simulink model "simulation"  (R2024a)
settings: Solver=FixedStepAuto  StartTime=0.0  StopTime=100  FixedStep=ts  RelTol=1e-3
values from neighbouring files (symbols this model uses):
  C = [0, 0, 1, 0, 0, 0 ... (first row only)    [setup.m]
  Ig = 10*(m*l^2)/3    (= 6)    [setup.m]
  m = 5    [setup.m]
  ni_r = 1    [setup.m]
  ni_x = 1    [setup.m]
  ni_y = 6    [setup.m]
  u_eq = [m*g; 0]    [setup.m]
  w = [1,      1 ... (first row only)    [setup.m]
  z_eq = z_init    [setup.m]
  z_init = [0;0;0;0;0;0]    [setup.m]
libraries: slpidlib x3, simulink x2
settings Model: Creator=enead  LastModifiedBy=enead
settings SolverCC: EnableFixedStepZeroCrossing=on
settings OptimizationCC: ReuseModelBlockBuffer=off
settings RTWCC: GPUComputeCapability=3.5

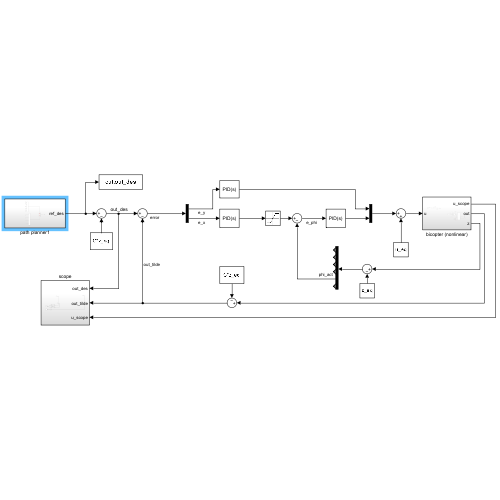
[thumbnail: Simulink's stored preview of the top-level diagram]
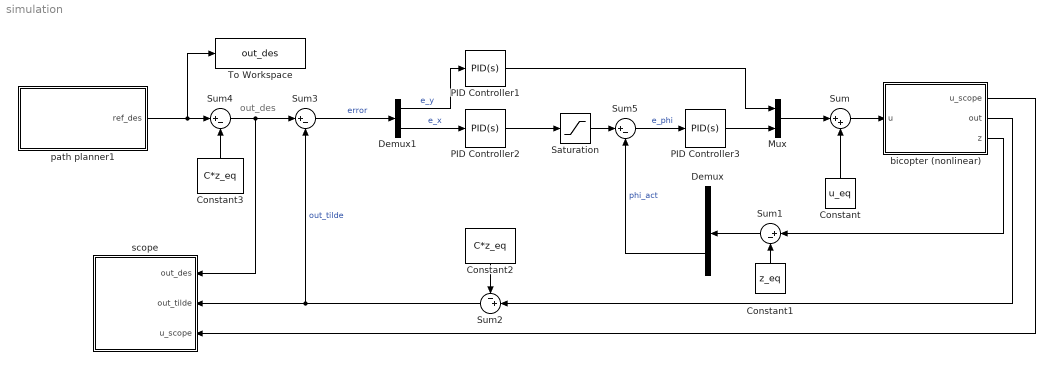
== system simulation ==
  note: out_des
  Constant : Constant  Value=u_eq
  Constant1 : Constant  Value=z_eq
  Constant2 : Constant  Value=C*z_eq
  Constant3 : Constant  Value=C*z_eq
  Demux : Demux  Outputs=6
  Demux1 : Demux  Outputs=2
  Mux : Mux  Inputs=2
  PID Controller1 : slpidlib/PID Controller  Controller=PID  Form=Parallel  TimeDomain=Continuous-time  UseExternalTs=off  SampleTime=-1  IntegratorMethod=Forward Euler  FilterMethod=Forward Euler  ControllerParametersSource=internal  P=10  I=0  UseKiTs=off  D=10  UseExternalDerivativeSource=off  N=20  UseFilter=on  TunerSelectOption=Transfer Function Based (PID Tuner App)  InitialConditionSource=internal  InitialConditionForIntegrator=0  InitialConditionForFilter=0  DifferentiatorICPrevScaledInput=0  ExternalReset=none  TrackingMode=off  Kt=1  LimitOutput=off  SatLimitsSource=internal  UpperSaturationLimit=inf  LowerSaturationLimit=-inf  LinearizeAsGain=on  AntiWindupMode=none  Kb=1  LimitIntegrator=off  UpperIntegratorSaturationLimit=inf  LowerIntegratorSaturationLimit=-inf  POutMin=[]  POutMax=[]  IOutMin=[]  IOutMax=[]  DOutMin=[]  DOutMax=[]  NOutMin=[]  NOutMax=[]  SumOutMin=[]  SumOutMax=[]  SaturationOutMin=[]  SaturationOutMax=[]  PParamMin=[]  PParamMax=[]  IParamMin=[]  IParamMax=[]  DParamMin=[]  DParamMax=[]  NParamMin=[]  NParamMax=[]  KbParamMin=[]  KbParamMax=[]  KtParamMin=[]  KtParamMax=[]  KbOutMin=[]  KbOutMax=[]  KtOutMin=[]  KtOutMax=[]  IntegratorOutMin=[]  IntegratorOutMax=[]  FilterOutMin=[]  FilterOutMax=[]  SumI1OutMin=[]  SumI1OutMax=[]  SumI2OutMin=[]  SumI2OutMax=[]  SumI3OutMin=[]  SumI3OutMax=[]  SumI4OutMin=[]  SumI4OutMax=[]  SumDOutMin=[]  SumDOutMax=[]  DifferentiatorOutMin=[]  DifferentiatorOutMax=[]  FilterDiffOutCoefMin=[]  FilterDiffOutCoefMax=[]  ReciprocalOutMin=[]  ReciprocalOutMax=[]  SumDenOutMin=[]  SumDenOutMax=[]  SumNumOutMin=[]  SumNumOutMax=[]  DivideOutMin=[]  DivideOutMax=[]  UdiffTsProdOutMin=[]  UdiffTsProdOutMax=[]  NTsProdOutMin=[]  NTsProdOutMax=[]  UintegralTsProdOutMin=[]  UintegralTsProdOutMax=[]  UngainTsProdOutMin=[]  UngainTsProdOutMax=[]  ClampingZeroOutDataTypeStr=Inherit: Inherit via back propagation  ClampingZeroOutMin=[]  ClampingZeroOutMax=[]  FilterDenConstantOutDataTypeStr=Inherit: Inherit via back propagation  FilterDenConstantOutMin=[]  FilterDenConstantOutMax=[]  PCopyOutDataTypeStr=Inherit: Inherit via back propagation  PCopyOutMin=[]  PCopyOutMax=[]  NCopyOutDataTypeStr=Inherit: Inherit via back propagation  NCopyOutMin=[]  NCopyOutMax=[]  IntegratorContinuousStateAttributes=''  IntegratorStateMustResolveToSignalObject=off  IntegratorRTWStateStorageClass=Auto  FilterContinuousStateAttributes=''  FilterStateMustResolveToSignalObject=off  FilterRTWStateStorageClass=Auto  ParallelPVariant=InternalParameters  IdealPVariant=Disabled  IVariant=InternalParameters  DVariant=InternalParameters  IntegratorVariant=Continuous  SatVariant=Disabled  AWVariant=Passthrough  PCopyVariant=Disabled  TRVariant=Disabled  FdbkBlocksVariant=Forward  IdealPFdbkVariant=Disabled  SatFdbkVariant=Disabled  DerivativeFilterVariant=ContFilter  NVariant=InternalParameters  NCopyVariant=Disabled  FilterICVariant=InternalICsFilter  IntegratorICVariant=InternalICs  ExternalResetVariant=Disabled  TRSumVariant=Passthrough  SumFdbkVariant=Disabled  SumVariant=Sum_PID  TsampFilterVariant=InternalTs  TsampNgainVariant=Passthrough  TsampIntegralVariant=Disabled_SignalSpec  ExternalSaturationOutDataTypeStr=Inherit: Same as second input  DerivativeSourceVariant=ErrorSignal
  PID Controller2 : slpidlib/PID Controller  Controller=PID  Form=Parallel  TimeDomain=Continuous-time  UseExternalTs=off  SampleTime=-1  IntegratorMethod=Forward Euler  FilterMethod=Forward Euler  ControllerParametersSource=internal  P=-0.07  I=0  UseKiTs=off  D=-0.07  UseExternalDerivativeSource=off  N=10  UseFilter=on  TunerSelectOption=Transfer Function Based (PID Tuner App)  InitialConditionSource=internal  InitialConditionForIntegrator=0  InitialConditionForFilter=0  DifferentiatorICPrevScaledInput=0  ExternalReset=none  TrackingMode=off  Kt=1  LimitOutput=off  SatLimitsSource=internal  UpperSaturationLimit=inf  LowerSaturationLimit=-inf  LinearizeAsGain=on  AntiWindupMode=none  Kb=1  LimitIntegrator=off  UpperIntegratorSaturationLimit=inf  LowerIntegratorSaturationLimit=-inf  POutMin=[]  POutMax=[]  IOutMin=[]  IOutMax=[]  DOutMin=[]  DOutMax=[]  NOutMin=[]  NOutMax=[]  SumOutMin=[]  SumOutMax=[]  SaturationOutMin=[]  SaturationOutMax=[]  PParamMin=[]  PParamMax=[]  IParamMin=[]  IParamMax=[]  DParamMin=[]  DParamMax=[]  NParamMin=[]  NParamMax=[]  KbParamMin=[]  KbParamMax=[]  KtParamMin=[]  KtParamMax=[]  KbOutMin=[]  KbOutMax=[]  KtOutMin=[]  KtOutMax=[]  IntegratorOutMin=[]  IntegratorOutMax=[]  FilterOutMin=[]  FilterOutMax=[]  SumI1OutMin=[]  SumI1OutMax=[]  SumI2OutMin=[]  SumI2OutMax=[]  SumI3OutMin=[]  SumI3OutMax=[]  SumI4OutMin=[]  SumI4OutMax=[]  SumDOutMin=[]  SumDOutMax=[]  DifferentiatorOutMin=[]  DifferentiatorOutMax=[]  FilterDiffOutCoefMin=[]  FilterDiffOutCoefMax=[]  ReciprocalOutMin=[]  ReciprocalOutMax=[]  SumDenOutMin=[]  SumDenOutMax=[]  SumNumOutMin=[]  SumNumOutMax=[]  DivideOutMin=[]  DivideOutMax=[]  UdiffTsProdOutMin=[]  UdiffTsProdOutMax=[]  NTsProdOutMin=[]  NTsProdOutMax=[]  UintegralTsProdOutMin=[]  UintegralTsProdOutMax=[]  UngainTsProdOutMin=[]  UngainTsProdOutMax=[]  ClampingZeroOutDataTypeStr=Inherit: Inherit via back propagation  ClampingZeroOutMin=[]  ClampingZeroOutMax=[]  FilterDenConstantOutDataTypeStr=Inherit: Inherit via back propagation  FilterDenConstantOutMin=[]  FilterDenConstantOutMax=[]  PCopyOutDataTypeStr=Inherit: Inherit via back propagation  PCopyOutMin=[]  PCopyOutMax=[]  NCopyOutDataTypeStr=Inherit: Inherit via back propagation  NCopyOutMin=[]  NCopyOutMax=[]  IntegratorContinuousStateAttributes=''  IntegratorStateMustResolveToSignalObject=off  IntegratorRTWStateStorageClass=Auto  FilterContinuousStateAttributes=''  FilterStateMustResolveToSignalObject=off  FilterRTWStateStorageClass=Auto  ParallelPVariant=InternalParameters  IdealPVariant=Disabled  IVariant=InternalParameters  DVariant=InternalParameters  IntegratorVariant=Continuous  SatVariant=Disabled  AWVariant=Passthrough  PCopyVariant=Disabled  TRVariant=Disabled  FdbkBlocksVariant=Forward  IdealPFdbkVariant=Disabled  SatFdbkVariant=Disabled  DerivativeFilterVariant=ContFilter  NVariant=InternalParameters  NCopyVariant=Disabled  FilterICVariant=InternalICsFilter  IntegratorICVariant=InternalICs  ExternalResetVariant=Disabled  TRSumVariant=Passthrough  SumFdbkVariant=Disabled  SumVariant=Sum_PID  TsampFilterVariant=InternalTs  TsampNgainVariant=Passthrough  TsampIntegralVariant=Disabled_SignalSpec  ExternalSaturationOutDataTypeStr=Inherit: Same as second input  DerivativeSourceVariant=ErrorSignal
  PID Controller3 : slpidlib/PID Controller  Controller=PID  Form=Parallel  TimeDomain=Continuous-time  UseExternalTs=off  SampleTime=-1  IntegratorMethod=Forward Euler  FilterMethod=Forward Euler  ControllerParametersSource=internal  P=14  I=0  UseKiTs=off  D=24  UseExternalDerivativeSource=off  N=5  UseFilter=on  TunerSelectOption=Transfer Function Based (PID Tuner App)  InitialConditionSource=internal  InitialConditionForIntegrator=0  InitialConditionForFilter=0  DifferentiatorICPrevScaledInput=0  ExternalReset=none  TrackingMode=off  Kt=1  LimitOutput=off  SatLimitsSource=internal  UpperSaturationLimit=inf  LowerSaturationLimit=-inf  LinearizeAsGain=on  AntiWindupMode=none  Kb=1  LimitIntegrator=off  UpperIntegratorSaturationLimit=inf  LowerIntegratorSaturationLimit=-inf  POutMin=[]  POutMax=[]  IOutMin=[]  IOutMax=[]  DOutMin=[]  DOutMax=[]  NOutMin=[]  NOutMax=[]  SumOutMin=[]  SumOutMax=[]  SaturationOutMin=[]  SaturationOutMax=[]  PParamMin=[]  PParamMax=[]  IParamMin=[]  IParamMax=[]  DParamMin=[]  DParamMax=[]  NParamMin=[]  NParamMax=[]  KbParamMin=[]  KbParamMax=[]  KtParamMin=[]  KtParamMax=[]  KbOutMin=[]  KbOutMax=[]  KtOutMin=[]  KtOutMax=[]  IntegratorOutMin=[]  IntegratorOutMax=[]  FilterOutMin=[]  FilterOutMax=[]  SumI1OutMin=[]  SumI1OutMax=[]  SumI2OutMin=[]  SumI2OutMax=[]  SumI3OutMin=[]  SumI3OutMax=[]  SumI4OutMin=[]  SumI4OutMax=[]  SumDOutMin=[]  SumDOutMax=[]  DifferentiatorOutMin=[]  DifferentiatorOutMax=[]  FilterDiffOutCoefMin=[]  FilterDiffOutCoefMax=[]  ReciprocalOutMin=[]  ReciprocalOutMax=[]  SumDenOutMin=[]  SumDenOutMax=[]  SumNumOutMin=[]  SumNumOutMax=[]  DivideOutMin=[]  DivideOutMax=[]  UdiffTsProdOutMin=[]  UdiffTsProdOutMax=[]  NTsProdOutMin=[]  NTsProdOutMax=[]  UintegralTsProdOutMin=[]  UintegralTsProdOutMax=[]  UngainTsProdOutMin=[]  UngainTsProdOutMax=[]  ClampingZeroOutDataTypeStr=Inherit: Inherit via back propagation  ClampingZeroOutMin=[]  ClampingZeroOutMax=[]  FilterDenConstantOutDataTypeStr=Inherit: Inherit via back propagation  FilterDenConstantOutMin=[]  FilterDenConstantOutMax=[]  PCopyOutDataTypeStr=Inherit: Inherit via back propagation  PCopyOutMin=[]  PCopyOutMax=[]  NCopyOutDataTypeStr=Inherit: Inherit via back propagation  NCopyOutMin=[]  NCopyOutMax=[]  IntegratorContinuousStateAttributes=''  IntegratorStateMustResolveToSignalObject=off  IntegratorRTWStateStorageClass=Auto  FilterContinuousStateAttributes=''  FilterStateMustResolveToSignalObject=off  FilterRTWStateStorageClass=Auto  ParallelPVariant=InternalParameters  IdealPVariant=Disabled  IVariant=InternalParameters  DVariant=InternalParameters  IntegratorVariant=Continuous  SatVariant=Disabled  AWVariant=Passthrough  PCopyVariant=Disabled  TRVariant=Disabled  FdbkBlocksVariant=Forward  IdealPFdbkVariant=Disabled  SatFdbkVariant=Disabled  DerivativeFilterVariant=ContFilter  NVariant=InternalParameters  NCopyVariant=Disabled  FilterICVariant=InternalICsFilter  IntegratorICVariant=InternalICs  ExternalResetVariant=Disabled  TRSumVariant=Passthrough  SumFdbkVariant=Disabled  SumVariant=Sum_PID  TsampFilterVariant=InternalTs  TsampNgainVariant=Passthrough  TsampIntegralVariant=Disabled_SignalSpec  ExternalSaturationOutDataTypeStr=Inherit: Same as second input  DerivativeSourceVariant=ErrorSignal
  Saturation : Saturate  UpperLimit=2  LowerLimit=-2
  Sum : Sum  Inputs=|++
  Sum{1,3..5} (4 alike) : Sum  Inputs=|+-
  Sum2 : Sum  Inputs=-+|
  To Workspace : ToWorkspace  VariableName=out_des  SaveFormat=Timeseries  SampleTime=-1
  bicopter (nonlinear) : Subsystem
  path planner1 : Subsystem
  scope : Subsystem
  wires:
  Sum/1 -> bicopter (nonlinear)/1(u)
  bicopter (nonlinear)/2(out) -> Sum2/2
  Constant2/1 -> Sum2/1
  Constant/1 -> Sum/2
  Sum2/1 -> scope/2(out_tilde), Sum3/2  "out_tilde"
  Constant3/1 -> Sum4/2
  bicopter (nonlinear)/3(z) -> Sum1/1
  Constant1/1 -> Sum1/2
  Sum4/1 -> Sum3/1, scope/1(out_des)
  Sum1/1 -> Demux/1
  Demux/5 -> Sum5/2  "phi_act"
  Mux/1 -> Sum/1
  Sum3/1 -> Demux1/1  "error"
  Demux1/2 -> PID Controller2/1  "e_x"
  Sum5/1 -> PID Controller3/1  "e_phi"
  PID Controller1/1 -> Mux/1
  PID Controller2/1 -> Saturation/1
  Demux1/1 -> PID Controller1/1  "e_y"
  path planner1/1(ref_des) -> To Workspace/1, Sum4/1
  Saturation/1 -> Sum5/1
  PID Controller3/1 -> Mux/2
  bicopter (nonlinear)/1(u_scope) -> scope/3(u_scope)

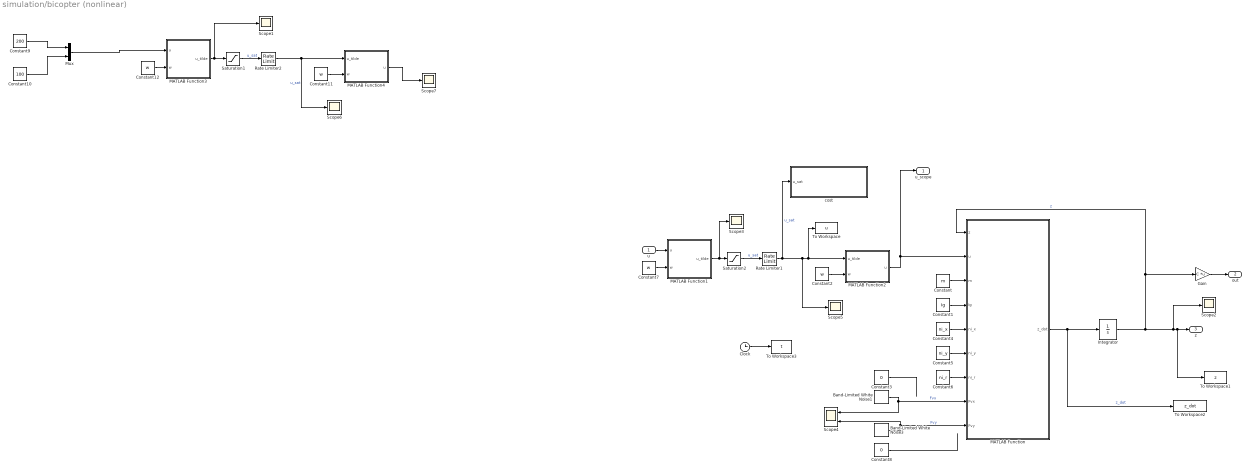
== system simulation/bicopter (nonlinear) ==
  u : Inport
  Band-Limited White Noise1 : simulink/Sources/Band-Limited White Noise  Cov=[7]  Ts=10  seed=[23341]
  Band-Limited White Noise3 : simulink/Sources/Band-Limited White Noise  Cov=[5]  Ts=15  seed=[23340]
  Clock : Clock
  Constant : Constant  Value=m
  Constant1 : Constant  Value=Ig
  Constant10 : Constant  Value=100
  Constant{2,7,11..12} (4 alike) : Constant  Value=w
  Constant3 : Constant  Value=0
  Constant4 : Constant  Value=ni_x
  Constant5 : Constant  Value=ni_y  VectorParams1D=off
  Constant6 : Constant  Value=ni_r
  Constant8 : Constant  Value=0
  Constant9 : Constant  Value=200
  Gain : Gain  Gain=C  Multiplication=Matrix(K*u)
  Integrator : Integrator  InitialCondition=z_init
  MATLAB Function : MATLAB Function  TreatAsAtomicUnit=on
  MATLAB Function1 : MATLAB Function  TreatAsAtomicUnit=on
  MATLAB Function2 : MATLAB Function  TreatAsAtomicUnit=on
  MATLAB Function3 : MATLAB Function  TreatAsAtomicUnit=on
  MATLAB Function4 : MATLAB Function  TreatAsAtomicUnit=on
  Mux : Mux  Inputs=2
  Rate Limiter1 : RateLimiter  RisingSlewLimit=25  FallingSlewLimit=-25  SampleTimeMode=inherited
  Rate Limiter2 : RateLimiter  RisingSlewLimit=25  FallingSlewLimit=-25  SampleTimeMode=inherited
  Saturation1 : Saturate  UpperLimit=30  LowerLimit=0
  Saturation2 : Saturate  UpperLimit=30  LowerLimit=0
  Scope{1..3,5..7} (6 alike) : Scope
  Scope4 : Scope  NumInputPorts=2
  To Workspace : ToWorkspace  VariableName=u  SaveFormat=Timeseries  SampleTime=-1
  To Workspace1 : ToWorkspace  VariableName=z  SaveFormat=Timeseries  SampleTime=-1
  To Workspace2 : ToWorkspace  VariableName=z_dot  SaveFormat=Timeseries  SampleTime=-1
  To Workspace3 : ToWorkspace  VariableName=t  SaveFormat=Timeseries  SampleTime=-1
  cost : Subsystem
  u_scope : Outport
  out : Outport  Port=2
  z : Outport  Port=3
  wires:
  Constant1/1 -> MATLAB Function/4(Ig)
  Integrator/1 -> Scope2/1, To Workspace1/1, z/1, Gain/1, MATLAB Function/1(z)  "z"
  Constant/1 -> MATLAB Function/3(m)
  MATLAB Function/1(z_dot) -> To Workspace2/1, Integrator/1  "z_dot"
  u/1 -> MATLAB Function1/1(u)
  Constant4/1 -> MATLAB Function/5(ni_x)
  Constant5/1 -> MATLAB Function/6(ni_y)
  Constant6/1 -> MATLAB Function/7(ni_r)
  MATLAB Function1/1(u_tilde) -> Saturation2/1, Scope3/1
  MATLAB Function2/1(u) -> u_scope/1, MATLAB Function/2(u)
  Constant2/1 -> MATLAB Function2/2(w)
  Constant7/1 -> MATLAB Function1/2(w)
  Clock/1 -> To Workspace3/1
  Gain/1 -> out/1
  Rate Limiter1/1 -> cost/1(u_sat), Scope5/1, To Workspace/1, MATLAB Function2/1(u_tilde)  "u_sat"
  Saturation2/1 -> Rate Limiter1/1  "u_sat"
  Band-Limited White Noise1/1 -> Scope4/1, MATLAB Function/8(Fvx)  "Fvx"
  Band-Limited White Noise3/1 -> MATLAB Function/9(Fvy), Scope4/2  "Fvy"
  Constant3/1 -> ?
  Constant8/1 -> ?
  Mux/1 -> MATLAB Function3/1(u)
  Constant9/1 -> Mux/1
  Constant10/1 -> Mux/2
  Rate Limiter2/1 -> Scope6/1, MATLAB Function4/1(u_tilde)  "u_sat"
  Constant11/1 -> MATLAB Function4/2(w)
  MATLAB Function3/1(u_tilde) -> Scope1/1, Saturation1/1
  Saturation1/1 -> Rate Limiter2/1  "u_sat"
  Constant12/1 -> MATLAB Function3/2(w)
  MATLAB Function4/1(u) -> Scope7/1

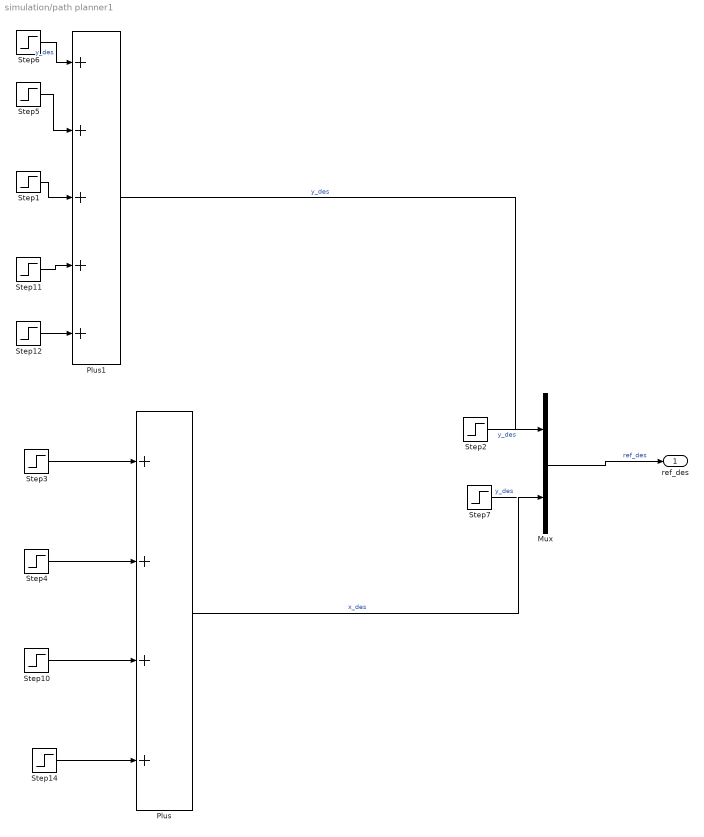
== system simulation/path planner1 ==
  Mux : Mux  Inputs=2
  Plus : Sum  Inputs=++++
  Plus1 : Sum  Inputs=+++++
  Step1 : Step  Time=15  After=-6.4  SampleTime=0
  Step10 : Step  Time=24  SampleTime=0
  Step11 : Step  Time=24  After=6.6  SampleTime=0
  Step12 : Step  Time=40  After=-6.9  SampleTime=0
  Step14 : Step  Time=31  After=-16  SampleTime=0
  Step2 : Step  After=3  SampleTime=0
  Step3 : Step  After=2  SampleTime=0
  Step4 : Step  Time=9  After=7.5  SampleTime=0
  Step5 : Step  Time=6  After=5.3  SampleTime=0
  Step6 : Step  After=2  SampleTime=0
  Step7 : Step  After=3  SampleTime=0
  ref_des : Outport
  wires:
  Mux/1 -> ref_des/1  "ref_des"
  Step6/1 -> Plus1/1  "y_des"
  Step3/1 -> Plus/1
  Step4/1 -> Plus/2
  Step5/1 -> Plus1/2
  Step1/1 -> Plus1/3
  Step10/1 -> Plus/3
  Plus1/1 -> Mux/1  "y_des"
  Plus/1 -> Mux/2  "x_des"
  Step12/1 -> Plus1/5
  Step11/1 -> Plus1/4
  Step14/1 -> Plus/4
  Step2/1 -> ?  "y_des"
  Step7/1 -> ?  "y_des"

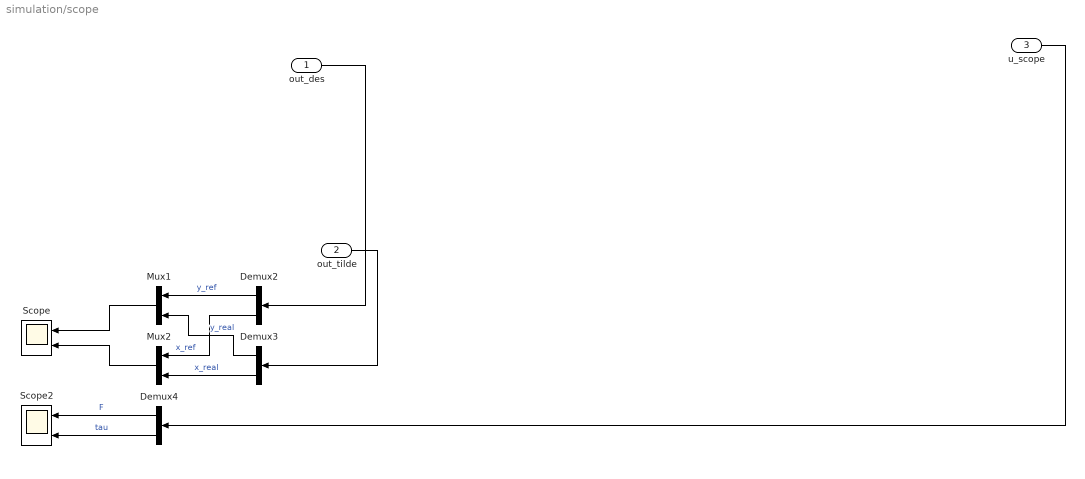
== system simulation/scope ==
  out_des : Inport
  out_tilde : Inport  Port=2
  u_scope : Inport  Port=3
  Demux2 : Demux  Outputs=2
  Demux3 : Demux  Outputs=2
  Demux4 : Demux  Outputs=2
  Mux1 : Mux  Inputs=2
  Mux2 : Mux  Inputs=2
  Scope : Scope  NumInputPorts=2
  Scope2 : Scope  NumInputPorts=2
  wires:
  Demux4/2 -> Scope2/2  "tau"
  Demux4/1 -> Scope2/1  "F"
  Demux2/2 -> Mux2/1  "x_ref"
  Mux2/1 -> Scope/2
  Mux1/1 -> Scope/1
  Demux3/2 -> Mux2/2  "x_real"
  Demux3/1 -> Mux1/2  "y_real"
  Demux2/1 -> Mux1/1  "y_ref"
  out_tilde/1 -> Demux3/1
  u_scope/1 -> Demux4/1
  out_des/1 -> Demux2/1

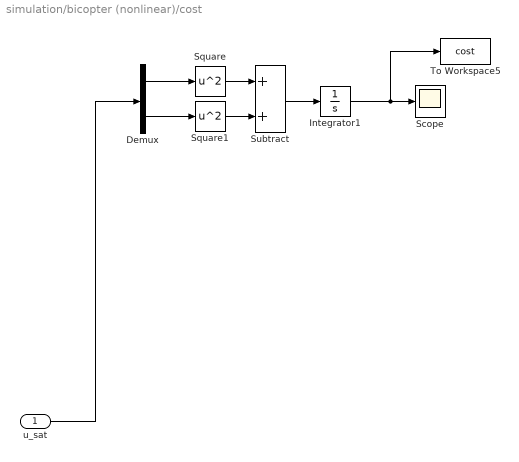
== system simulation/bicopter (nonlinear)/cost ==
  u_sat : Inport
  Demux : Demux  Outputs=2
  Integrator1 : Integrator
  Scope : Scope
  Square : Math  Operator=square
  Square1 : Math  Operator=square
  Subtract : Sum
  To Workspace5 : ToWorkspace  VariableName=cost  SaveFormat=Timeseries  SampleTime=-1
  wires:
  Integrator1/1 -> To Workspace5/1, Scope/1
  Square/1 -> Subtract/1
  Demux/2 -> Square1/1
  Square1/1 -> Subtract/2
  u_sat/1 -> Demux/1
  Subtract/1 -> Integrator1/1
  Demux/1 -> Square/1

== matlab function simulation/bicopter (nonlinear)/MATLAB Function ==
  data: z input; u input; z_dot output; m input; Ig input; ni_x input; ni_y input; ni_r input; Fvx input; Fvy input
function z_dot = drone_nonlinear_evol(z, u, m, Ig, ni_x, ni_y, ni_r, Fvx, Fvy)

    g = 9.81;

    x = z(1);
    x_dot = z(2);
    y = z(3);
    y_dot = z(4);
    phi = z(5);
    phi_dot = z(6);

    F = u(1);
    tau = u(2);

    z_dot1 = x_dot;
    z_dot2 = - F/m * sin(phi) - ni_x*x_dot*sin(phi)/m - Fvx/m;
    z_dot3 = y_dot;
    z_dot4 = F/m * cos(phi) - g  - ni_y*y_dot*cos(phi)/m - Fvy/m;
    z_dot5 = phi_dot;
    z_dot6 = tau/Ig - ni_r*phi_dot/Ig;

    z_dot = [z_dot1; z_dot2; z_dot3; z_dot4; z_dot5; z_dot6];

== matlab function simulation/bicopter (nonlinear)/MATLAB Function1 ==
  data: u input; u_tilde output; w input
function u_tilde = tilding(u, w)

    u_tilde = w\u;

== matlab function simulation/bicopter (nonlinear)/MATLAB Function2 ==
  data: u_tilde input; u output; w input
function u = detilding(u_tilde, w)

    u = w*u_tilde;

== matlab function simulation/bicopter (nonlinear)/MATLAB Function3 ==
  data: u input; u_tilde output; w input
function u_tilde = tilding(u, w)

    u_tilde = w\u;

== matlab function simulation/bicopter (nonlinear)/MATLAB Function4 ==
  data: u_tilde input; u output; w input
function u = detilding(u_tilde, w)

    u = w*u_tilde;
